simulink model "car4"  (R2016a)
settings: Solver=VariableStepAuto  StartTime=0.0  StopTime=20  RelTol=1e-3
undefined symbols (not defined in the file or in its folder): sigbuilder_block
libraries: simulink x1
settings Model: Creator=richa  LastModifiedBy=richa

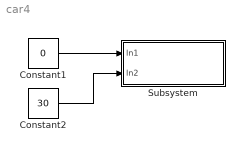
== system car4 ==
  Constant1 : Constant  Value=0
  Constant2 : Constant  Value=30
  Subsystem : Subsystem
  wires:
  Constant1/1 -> Subsystem/1(In1)
  Constant2/1 -> Subsystem/2(In2)

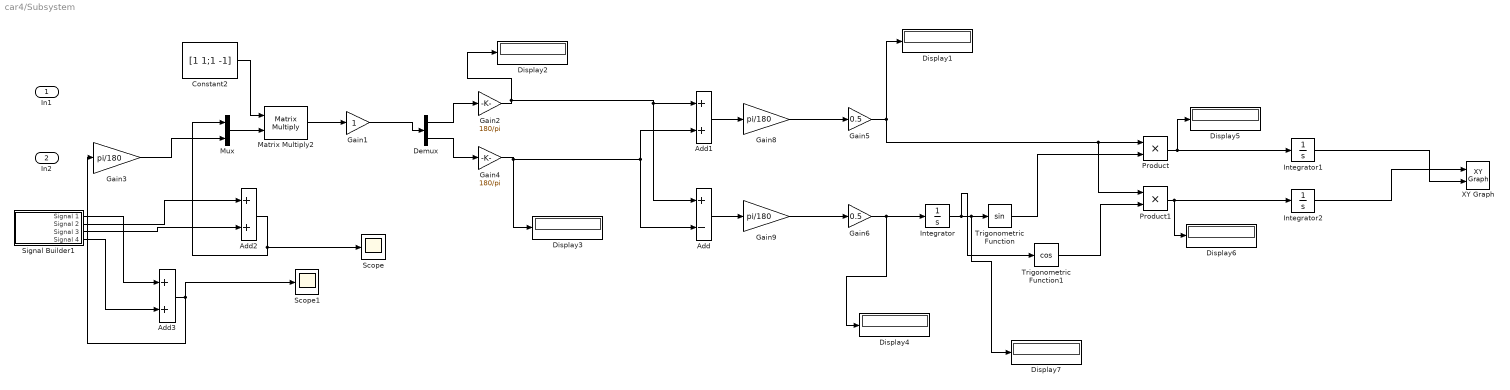
== system car4/Subsystem ==
  In1 : Inport
  In2 : Inport  Port=2
  Add : Sum  Inputs=+-
  Add1 : Sum
  Add2 : Sum
  Add3 : Sum
  Constant2 : Constant  Value=[1 1;1 -1]
  Demux : Demux  Outputs=2
  Display{1..7} (7 alike) : Display
  Gain1 : Gain
  Gain2 : Gain  Gain=180/pi
  Gain3 : Gain  Gain=pi/180
  Gain4 : Gain  Gain=180/pi
  Gain5 : Gain  Gain=0.5
  Gain6 : Gain  Gain=0.5
  Gain8 : Gain  Gain=pi/180
  Gain9 : Gain  Gain=pi/180
  Integrator : Integrator
  Integrator1 : Integrator
  Integrator2 : Integrator
  Matrix Multiply2 : Product  Multiplication=Matrix(*)
  Mux : Mux  Inputs=2
  Product : Product
  Product1 : Product
  Scope : Scope
  Scope1 : Scope
  Signal Builder1 : Subsystem  Tag=STV Subsys  LoadFcn=sigbuilder_block('load',[26 198 550.5 400 ]);  StartFcn=sigbuilder_block('start');  StopFcn=sigbuilder_block('stop');  ClipboardFcn=sigbuilder_block('clipboard');  mask(Sigbuilder block){}
      mask help: Simulink:masks:SigbuilderBlock_MD
      mask init:
      | if ~strcmp(get_param(bdroot(gcbh),'SimulationStatus'),'stopped') tuvar = sigbuilder_block('maskInit'); end
      settings: CopyFcn=sigbuilder_block('copy');  DeleteFcn=sigbuilder_block('delete');  ModelCloseFcn=sigbuilder_block('modelClose');  PreSaveFcn=sigbuilder_block('preSave');  PauseFcn=sigbuilder_block('pause');  ContinueFcn=sigbuilder_block('continue');  NameChangeFcn=sigbuilder_block('namechange');  OpenFcn=sigbuilder_block('open',[437.6 199.2 550.4 400 ]);  CloseFcn=sigbuilder_block('close');
      mask Display: plot(0, 0, 100, 100,[2, 2, 32, 32, 2], [68, 8, 8, 68, 68],[32, 2], [38, 38], [32, 19, 2],[53, 60, 44], [32, 17, 17, 2],[16, 16, 31, 31]);txt = getActiveGroup(gcbh);text(2, 100, txt,'verticalAlignment', 'top');
  Trigonometric Function : Trigonometry  ApproximationMethod=CORDIC
  Trigonometric Function1 : Trigonometry  Operator=cos  ApproximationMethod=CORDIC
  XY Graph : simulink/Sinks/XY Graph  xmin=-10  xmax=10  ymin=-10  ymax=10  st=0
  wires:
  Mux/1 -> Matrix Multiply2/2
  Gain1/1 -> Demux/1
  Demux/1 -> Gain2/1
  Gain3/1 -> Mux/2
  Demux/2 -> Gain4/1
  Constant2/1 -> Matrix Multiply2/1
  Matrix Multiply2/1 -> Gain1/1
  Gain2/1 -> Add/1, Add1/1, Display2/1
  Gain4/1 -> Display3/1, Add/2, Add1/2
  Gain5/1 -> Product1/1, Product/1, Display1/1
  Gain6/1 -> Integrator/1, Display4/1
  Add1/1 -> Gain8/1
  Add/1 -> Gain9/1
  Gain8/1 -> Gain5/1
  Gain9/1 -> Gain6/1
  Integrator/1 -> Trigonometric Function1/1, Display7/1, Trigonometric Function/1
  Trigonometric Function/1 -> Product/2
  Trigonometric Function1/1 -> Product1/2
  Product/1 -> Integrator1/1, Display5/1
  Product1/1 -> Integrator2/1, Display6/1
  Integrator2/1 -> XY Graph/1
  Integrator1/1 -> XY Graph/2
  Signal Builder1/2(Signal 2) -> Add2/1
  Add2/1 -> Scope/1, Mux/1
  Add3/1 -> Gain3/1, Scope1/1
  Signal Builder1/1(Signal 1) -> Add3/1
  Signal Builder1/4(Signal 4) -> Add3/2
  Signal Builder1/3(Signal 3) -> Add2/2

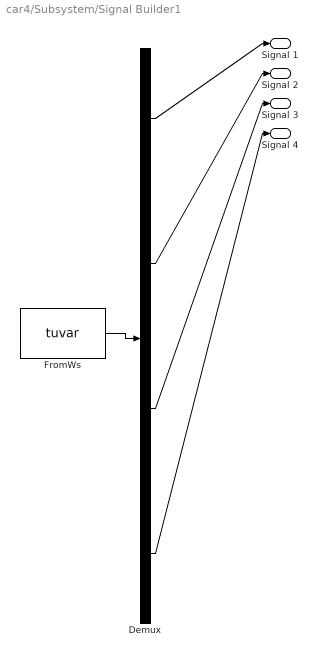
== system car4/Subsystem/Signal Builder1 ==
  Demux : Demux  Tag=STV Demux
  FromWs : FromWorkspace  Tag=STV FromWs  VariableName=tuvar  SampleTime=0
      SigBuilderData=|
      | common.afterFinalStr = 'Extrapolate'
      | common.sampleTime = 0
      | dataSet.timeRange = [0 10]
      | dataSet.name = 'Group 1'
      | sbobj.Groups.Name = 'Group 1'
      | sbobj.Groups.Signals(1).Name = 'Signal 1'
      | sbobj.Groups.Signals(1).XData = [0 2 2 4.02 4.02 10]
      | sbobj.Groups.Signals(1).YData = [0 0 46 46 0 0]
      | sbobj.Groups.Signals(2).Name = 'Signal 2'
      | sbobj.Groups.Signals(2).XData = [0 2.04 2.04 10]
      | sbobj.Groups.Signals(2).YData = [1 1 0 0]
      | sbobj.Groups.Signals(3).Name = 'Signal 3'
      | sbobj.Groups.Signals(3).XData = [0 6.66 6.66 7.8 7.8 10]
      | sbobj.Groups.Signals(3).YData = [0 0 1.11 1.11 0 0]
      | sbobj.Groups.Signals(4).Name = 'Signal 4'
      | sbobj.Groups.Signals(4).XData = [0 5.44 5.44 6.36 6.36 10]
      | sbobj.Groups.Signals(4).YData = [0 0 35.8 35.8 0 0]
  Signal 1 : Outport  Tag=STV Outport
  Signal 2 : Outport  Tag=STV Outport  Port=2
  Signal 3 : Outport  Tag=STV Outport  Port=3
  Signal 4 : Outport  Tag=STV Outport  Port=4
  wires:
  FromWs/1 -> Demux/1
  Demux/1 -> Signal 1/1
  Demux/2 -> Signal 2/1
  Demux/3 -> Signal 3/1
  Demux/4 -> Signal 4/1
